simulink model "test_firs"  (Simulink 6.2)
settings: Solver=ode45  StartTime=0.0  StopTime=500  RelTol=1e-3
undefined symbols (not defined in the file or in its folder): now, pfb_coefs
libraries: xbsIndex_r3 x151, pfb_library x1, simulink x1
(part 1 of 3)
settings Model: LastModifiedBy=mdexter
settings DebuggingCC: SolverPrmCheckMsg=warning

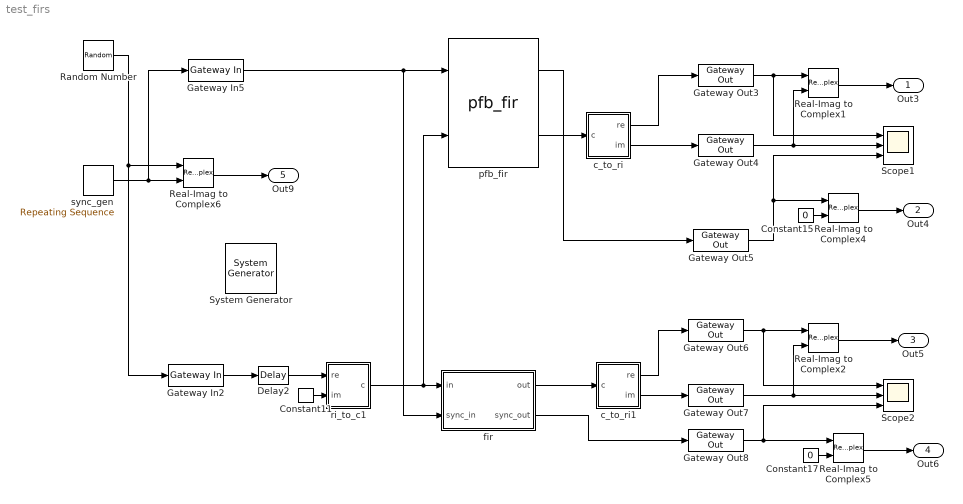
== system test_firs ==
  " System Generator" : xbsIndex_r3/ System Generator  Tag=genX  xilinxfamily=Virtex2  part=xc2v1000  speed=-4  package=bg575  synthesis_tool=XST  directory=./netlist  testbench=off  simulink_period=1  sysclk_period=100  incr_netlist=off  trim_vbits=Everywhere in SubSystem  dbl_ovrd=According to Block Masks  core_generation=According to Block Masks  run_coregen=off  deprecated_control=off  eval_field=0
      settings: AttributesFormatString=System\nGenerator
  Constant11 : xbsIndex_r3/Constant  const=0  equ=P=C  arith_type=Unsigned  n_bits=8  bin_pt=7  opselect=C  inp2=PCIN>>17  opr=+  inp1=P  carry=CIN  iostate=0  explicit_period=on  period=1  dbl_ovrd=off
  Constant15 : Constant  Value=0
  Constant17 : Constant  Value=0
  Delay2 : xbsIndex_r3/Delay  latency=1  reg_retiming=off  explicit_period=off  period=1  en=off  accept_only_valid=off  init_zero=on  dbl_ovrd=off  show_param=off
      settings: xl_area=[0, 0, 0, 0, 0, 0, 0]
  Gateway In2 : xbsIndex_r3/Gateway In  arith_type="Signed  (2's comp)"  n_bits=8  bin_pt=7  quantization="Round  (unbiased: +/- Inf)"  overflow=Wrap  period=1  timing_constraint=None  locs_specified=off  LOCs={}  needs_fixed_name=off  dbl_ovrd=off  show_param=off
      settings: xl_area=[0, 0, 0, 0, 0, 0, 0]
  Gateway In5 : xbsIndex_r3/Gateway In  arith_type=Boolean  n_bits=8  bin_pt=7  quantization=Truncate  overflow=Wrap  period=1  timing_constraint=None  locs_specified=off  LOCs={}  needs_fixed_name=off  dbl_ovrd=off  show_param=off
      settings: xl_area=[0, 0, 0, 0, 0, 0, 0]
  Gateway Out{3..8} (6 alike) : xbsIndex_r3/Gateway Out  output_type=Double  nbits=8  bin_pt=6  arith_type=Boolean  quantization=Truncate  overflow=Wrap  hdl_port=on  timing_constraint=None  locs_specified=off  LOCs={}  needs_fixed_name=off  show_param=off
      settings: xl_area=[0, 0, 0, 0, 0, 0, 0]
  Random Number : RandomNumber  Variance=.3^2  Seed=floor(100*(now-floor(now)))  SampleTime=1
  Real-Imag to Complex{1..2,4..6} (5 alike) : RealImagToComplex
  Scope1 : Scope  NumInputPorts=3
      settings: YMin=-5~-5~-5  YMax=5~5~5
  Scope2 : Scope  NumInputPorts=3
      settings: YMin=-5~-5~-5  YMax=5~5~5  SaveName=ScopeData2
  c_to_ri : Subsystem  mask(Complex to Real-Imag){n_bits=18, bin_pt=17}
      mask prompts: n_bits "Bit Width"; bin_pt "Binary Point"
      mask help: Outputs real and imaginary components of a complex input.
      mask init:
      | c_to_ri_init(gcb,n_bits,bin_pt);
      settings: AttributesFormatString=18_17 r/i
      mask Help:
      | <pre>
      | Description::
      | 
      | Outputs real and imaginary components of a complex input.
      | Useful for simplifying interconnects.
      | See also: Real-Imag to Complex (ri_to_c)
      | 
      | Mask Parameters::
      | 
      | Bit Width (n_bits): Specifies the width of the real/imaginary components.
      | Assumed equal for both components.
      | 
      | Binary Point (bin_pt): Specifies the binary point location in the real/imaginary components.
      | Assumed equal for both components.
      | </pre>
  c_to_ri1 : Subsystem  mask(Complex to Real-Imag){n_bits=9, bin_pt=7}
      mask prompts: n_bits "Bit Width"; bin_pt "Binary Point"
      mask help: Outputs real and imaginary components of a complex input.
      mask init:
      | c_to_ri_init(gcb,n_bits,bin_pt);
      settings: AttributesFormatString=9_7 r/i
      mask Help:
      | <pre>
      | Description::
      | 
      | Outputs real and imaginary components of a complex input.
      | Useful for simplifying interconnects.
      | See also: Real-Imag to Complex (ri_to_c)
      | 
      | Mask Parameters::
      | 
      | Bit Width (n_bits): Specifies the width of the real/imaginary components.
      | Assumed equal for both components.
      | 
      | Binary Point (bin_pt): Specifies the binary point location in the real/imaginary components.
      | Assumed equal for both components.
      | </pre>
  fir : Subsystem  AncestorBlock=newfft_library/FIR/fir  mask(FIR Filter){coefs=pfb_coefs(64,4), n_bits_c=9, bin_pt_c=8, n_bits_d=8, bin_pt_d=7, n_bits_o=9, bin_pt_o=7, coef_bram=on, delay_bram=on, mult_latency=3, add_latency=1, show_sbo=on, munge_submasks=DumbDown}
      mask prompts: coefs "Tap Coefficients"; n_bits_c "Number of Coefficient Bits"; bin_pt_c "Coefficient Binary Point"; n_bits_d "Number of Data Bits"; bin_pt_d "Data Binary Point"; n_bits_o "Number of Bits Out"; bin_pt_o "Binary Point Out"; coef_bram "Use BRAM for Coefficients"; delay_bram "Use BRAM for Delay"; mult_latency "Multiplier Latency"; add_latency "Adder Latency"; show_sbo "Show Sub-Block Options"; munge_submasks "Sub-Block Masks"
      mask help: A Finite Impluse Response Filter. This FIR filter does not have provisions for folding the input sequence to improve multiplier efficiency, so it is suboptimal for "regular" (i.e. non-WOLA) FIR filters. It is intended primarily for WOLA (Weighted OverLap Add) FIR filters.
      mask init:
      | tic
      | fir_init(gcb, ...
      |   coefs, ...
      |   n_bits_c, ...
      |   bin_pt_c, ...
      |   n_bits_d, ...
      |   bin_pt_d, ...
      |   n_bits_o, ...
      |   bin_pt_o, ...
      |   coef_bram, ...
      |   delay_bram, ...
      |   mult_latency, ...
      |   add_latency, ...
      |   lower(get_param(gcb,'munge_submasks')) );
      | disp('fir_init complete.');
      | toc
      settings: AttributesFormatString=|
      | 4 taps
      | 9_8 coefs
      | 8_7 in
      | 9_7 out
      mask Help:
      | <pre>
      | Description::
      | 
      | A Finite Impluse Response Filter.
      | 
      | This Finite Impluse Response Filter does not have provisions for folding the input
      | sequence to improve multiplier efficiency, so it is suboptimal for "regular" (i.e. non-WOLA)
      | FIR filters.  It is intended primarily for WOLA (Weighted OverLap Add) FIR filters.
      | 
      | Mask Parameters::
      | 
      | Coefficiant(s) (coefs): Matrix of real double(s) to use as coefficient(s).
      | One column per tap.  Multiple rows will create a WOLA filter.
      | These should be specified as doubles.  They will be rounded/saturated according to the
      | specified number of bits (n_bits_c) and binary point (bin_pt_c).
      | 
      | Number of Coefficient Bits (n_bits_c): The number of bits used for the fixed point binary
      | representation of the coefficient(s).
      | 
      | Coefficient Binary Point (bin_pt_c): The binary point of the fixed point binary representation
      | of the coefficient(s).
      | 
      | Number of Data Bits (n_bits_d): The number of bits for real/imaginary components of the data.
      | 
      | Data Binary Point (bin_pt_d): The binary point for real/imaginary components of the data.
      | 
      | Number of Bits Out (n_bits_o): Specifies the width of the output (overflow wraps).
      | The internal adders will use a bit width of (n_bits_o-bin_pt_o+bin_pt_c+bin_pt_d).
      | 
      | Binary Point Out (bin_pt_o): Specifies the binary point of the output (quantization truncates).
      | The internal adders will use a binary point of (bin_pt_c+bin_pt_d).
      | 
      | Use BRAM for Coefficients (coef_bram): Check this checkbox to store the coefficients in BRAM.
      | If unchecked, the coefficients will be stored in distributed memory (i.e. slices).
      | This is only relevant is length(coef) is greater than 1; otherwise, a constant block is used.
      | 
      | Use BRAM for Delay (delay_bram): Check this checkbox to implement the delay using BRAM.
      | If unchecked, the delay will be implemented using SLR16 elements (i.e. slices).
      | 
      | Multiplier Latency (mult_latency): Latency to use for the underlying multiplier.
      | 
      | Adder Latency (add_latency): Latency to use for the underlying adder.
      | </pre>
      mask StyleString: edit,edit,edit,edit,edit,edit,edit,checkbox,checkbox,edit,edit,checkbox,popup(Keep|DumbDown|Unmask)
      mask CallbackString:
      | |||||||||||mvs=get_param(gcb,'MaskVisibilityString');
      | if strcmp(get_param(gcb,'show_sbo'),'on')
      |   onoff='on';
      | else
      |   onoff='off';
      | end
      | mvs=regexprep(mvs,'o[nf]*$',onoff);
      | set_param(gcb,'MaskVisibilityString',mvs);
      | |
  pfb_fir : pfb_library/pfb_fir  PFBSize=6  TotalTaps=4  WindowType=hamming  n_inputs=0  MakeBiplex=off  BitWidthIn=8  BitWidthOut=18  CoeffBitWidth=9  CoeffDistMem=off  add_latency=1  mult_latency=3  bram_latency=1  quantization="Round  (unbiased: Even Values)"  fwidth=1
      link override pol1_in1_first_tap/sync_delay/Constant: equ=P=C
      link override pol1_in1_first_tap/sync_delay/Constant1: equ=P=C
      link override pol1_in1_first_tap/sync_delay/Constant2: equ=P=C
      link override pol1_in1_first_tap/sync_delay/Constant3: equ=P=C
      link override pol1_in1_tap2/sync_delay/Constant: equ=P=C
      link override pol1_in1_tap2/sync_delay/Constant1: equ=P=C
      link override pol1_in1_tap2/sync_delay/Constant2: equ=P=C
      link override pol1_in1_tap2/sync_delay/Constant3: equ=P=C
      link override pol1_in1_tap3/sync_delay/Constant: equ=P=C
      link override pol1_in1_tap3/sync_delay/Constant1: equ=P=C
      link override pol1_in1_tap3/sync_delay/Constant2: equ=P=C
      link override pol1_in1_tap3/sync_delay/Constant3: equ=P=C
  ri_to_c1 : Subsystem  mask(Real-Imag to Complex){}
      mask help: Concatenates real and imaginary inputs into a complex output.
      mask init:
      | ri_to_c_init(gcb);
      mask Help:
      | <pre>
      | Description::
      | 
      | Concatenates a real and imaginary input into a complex output.
      | Useful for simplifying interconnects.
      | See also: Complex to Real-Imag (c_to_ri)
      | 
      | Mask Parameters::
      | 
      | (N/A)
      | </pre>
  sync_gen : simulink/Sources/Repeating Sequence  rep_seq_t=[0:64]  rep_seq_y=[1 zeros(1,63) 1]
  Out3 : Outport
  Out4 : Outport  Port=2
  Out5 : Outport  Port=3
  Out6 : Outport  Port=4
  Out9 : Outport  Port=5
  wires:
  Random Number/1 -> Real-Imag to Complex6/1, Gateway In2/1
  Gateway Out3/1 -> Scope1/1, Real-Imag to Complex1/1
  Gateway Out4/1 -> Scope1/2, Real-Imag to Complex1/2
  Gateway Out5/1 -> Scope1/3, Real-Imag to Complex4/1
  Gateway In5/1 -> fir/2(sync_in), pfb_fir/1
  Gateway In2/1 -> Delay2/1
  Gateway Out6/1 -> Real-Imag to Complex2/1, Scope2/1
  Gateway Out7/1 -> Scope2/2, Real-Imag to Complex2/2
  Gateway Out8/1 -> Scope2/3, Real-Imag to Complex5/1
  fir/2(sync_out) -> Gateway Out8/1
  fir/1(out) -> c_to_ri1/1(c)
  c_to_ri/2(im) -> Gateway Out4/1
  ri_to_c1/1(c) -> fir/1(in), pfb_fir/2
  Constant11/1 -> ri_to_c1/2(im)
  sync_gen/1 -> Real-Imag to Complex6/2, Gateway In5/1
  Delay2/1 -> ri_to_c1/1(re)
  c_to_ri/1(re) -> Gateway Out3/1
  Real-Imag to Complex1/1 -> Out3/1
  c_to_ri1/1(re) -> Gateway Out6/1
  c_to_ri1/2(im) -> Gateway Out7/1
  Real-Imag to Complex2/1 -> Out5/1
  Real-Imag to Complex4/1 -> Out4/1
  Real-Imag to Complex5/1 -> Out6/1
  Constant15/1 -> Real-Imag to Complex4/2
  Constant17/1 -> Real-Imag to Complex5/2
  Real-Imag to Complex6/1 -> Out9/1
  pfb_fir/1 -> Gateway Out5/1
  pfb_fir/2 -> c_to_ri/1(c)

== system test_firs/c_to_ri ==
  c : Inport  Port=1  LatchInput=off
  force_im : xbsIndex_r3/Reinterpret  force_arith_type=on  arith_type="Signed  (2's comp)"  force_bin_pt=on  bin_pt=17  force_valid=on
  force_re : xbsIndex_r3/Reinterpret  force_arith_type=on  arith_type="Signed  (2's comp)"  force_bin_pt=on  bin_pt=17  force_valid=on
  slice_im : xbsIndex_r3/Slice  mode=Lower Bit Location + Width  nbits=18  bit1=0  base1=MSB of Input  bit0=0  base0=LSB of Input  boolean_output=off  explicit_period=off  period=1  dbl_ovrd=off
  slice_re : xbsIndex_r3/Slice  mode=Upper Bit Location + Width  nbits=18  bit1=0  base1=MSB of Input  bit0=0  base0=LSB of Input  boolean_output=off  explicit_period=off  period=1  dbl_ovrd=off
  re : Outport
  im : Outport  Port=2
  wires:
  slice_re/1 -> force_re/1
  slice_im/1 -> force_im/1
  force_re/1 -> re/1
  force_im/1 -> im/1
  c/1 -> slice_re/1, slice_im/1

== system test_firs/c_to_ri1 ==
  c : Inport  Port=1  LatchInput=off
  force_im : xbsIndex_r3/Reinterpret  force_arith_type=on  arith_type="Signed  (2's comp)"  force_bin_pt=on  bin_pt=7  force_valid=on
  force_re : xbsIndex_r3/Reinterpret  force_arith_type=on  arith_type="Signed  (2's comp)"  force_bin_pt=on  bin_pt=7  force_valid=on
  slice_im : xbsIndex_r3/Slice  mode=Lower Bit Location + Width  nbits=9  bit1=0  base1=MSB of Input  bit0=0  base0=LSB of Input  boolean_output=off  explicit_period=off  period=1  dbl_ovrd=off
  slice_re : xbsIndex_r3/Slice  mode=Upper Bit Location + Width  nbits=9  bit1=0  base1=MSB of Input  bit0=0  base0=LSB of Input  boolean_output=off  explicit_period=off  period=1  dbl_ovrd=off
  re : Outport
  im : Outport  Port=2
  wires:
  c/1 -> slice_im/1, slice_re/1
  force_im/1 -> im/1
  force_re/1 -> re/1
  slice_im/1 -> force_im/1
  slice_re/1 -> force_re/1

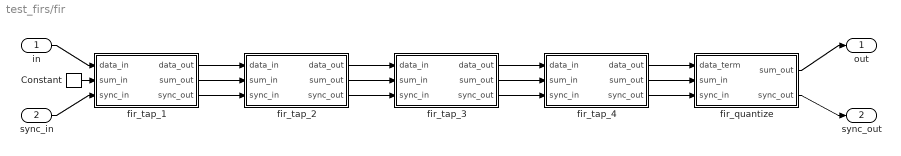
== system test_firs/fir ==
  in : Inport  Port=1  LatchInput=off
  sync_in : Inport  Port=2  LatchInput=off
  Constant : xbsIndex_r3/Constant  const=0  equ=P=C  arith_type=Unsigned  n_bits=34  bin_pt=0  opselect=C  inp2=PCIN>>17  opr=+  inp1=P  carry=CIN  iostate=0  explicit_period=on  period=1  dbl_ovrd=off
  fir_quantize : Subsystem  mask(FIR Filter Quantizer){n_bits_s=17, bin_pt_s=15, n_bits_o=9, bin_pt_o=7}
      mask prompts: n_bits_s "Number of Bits In"; bin_pt_s "Binary Point In"; n_bits_o "Number of Bits Out"; bin_pt_o "Binary Point Out"
      mask help: A Finite Impluse Response Filter ouput quantizer. This FIR filter output quantizer rounds the sum_in value to the precision specified by n_bits and bin_pt. Overflow wraps, but quantization rounds to even if input binary point is greater than output binary point, otherwise quantization tuncates.
      settings: AttributesFormatString=|
      | 17_15 in
      | 9_7 out
      | round even
      mask Help:
      | <pre>
      | Description::
      | 
      | A Finite Impluse Response Filter ouput quantizer.  This FIR filter output quantizer
      | rounds the sum_in value to the precision specified by n_bits and bin_pt.
      | 
      | Overflow wraps, but quantization rounds to even if input binary point is greater
      | than output binary point, otherwise quantization tuncates.
      | 
      | Mask Parameters::
      | 
      | Number of Bits In (n_bits_s): Specifies the width of the sum_in input.
      | 
      | Binary Point In (bin_pt_s): Specifies the binary point of the sum_in input.
      | 
      | Number of Bits Out (n_bits_o): Specifies the width of the output (overflow wraps).
      | 
      | Binary Point Out (bin_pt_o): Specifies the binary point of the output (quantization rounds to even
      | if input binary point is greater than output binary point, othersie quantization truncates).
      | </pre>
  fir_tap_1 : Subsystem  mask(FIR Filter Tap (Real Coefficients)){delay=64, coef=[-0.00411973909604202;-0.0119015518843096;-0.0190818823895147;-0.0256724955662416;-0.03168654178132;-0.0371384687203353;-0.0420439301426944;-0.0464196919199395;-0.0502835357982813;-0.0536541613305752;-0.0565510864251856;-0.0589945469593747;-0.0610053959030371;-0.0626050023947942;-0.0638151512067052;-0.0646579430261756;-0.0651556959741166;-0.0653308487670656;-0.0652058659179099;-0.064803145355121;-0.0641449288240917;-0.063253215416367;-0.0621496785533557;-0.0608555867306188;-0.0593917283071436;-0.057778340601254;-0.0560350435310833;-0.0541807780129703;-0.0522337493058552;-0.050211375463868;-0.0481302410329562;-0.0460060561007039;-0.0438536207815986;-0.0416867951930131;-0.039518474950235;-0.0373605721821118;-0.035224002042413;-0.0331186746659681;-0.0310534924931389;-0.0290363528613422;-0.0270741557382724;-0.0251728164482839;-0.0233372832211883;-0.0215715593716044;-0.0198787298970449;-0.018260992264242;-0.0167196911358607;-0.0152553567738119;-0.0138677468409146;-0.0125558913097251;-0.0113181401759998;-0.0101522136645361;-0.00905525460705801;-0.00802388266542662;-0.0070542500687595;-0.0061420985300509;-0.00528281700660057;-0.00447149996896613;-0.00370300584524142;-0.00297201531120363;-0.00227308910223182;-0.00160072502983972;-0.000949413894136895;-0.000313693993479576], n_bits_c=9, bin_pt_c=8, n_bits_d=8, bin_pt_d=7, n_bits_s=17, bin_pt_s=15, coef_bram=on, delay_bram=on, mult_latency=3, add_latency=1, add_bypass=on}
      mask prompts: delay "Tap Delay"; coef "Tap Coefficient(s)"; n_bits_c "Number of Coefficient Bits"; bin_pt_c "Coefficient Binary Point"; n_bits_d "Number of Data Bits"; bin_pt_d "Data Binary Point"; n_bits_s "Number of Sum Bits"; bin_pt_s "Sum Binary Point"; coef_bram "Use BRAM for Coefficients"; delay_bram "Use BRAM for Delay"; mult_latency "Multiplier Latency"; add_latency "Adder Latency"; add_bypass "Bypass Adder"
      mask help: A Finite Impluse Response Filter tap with real coefficients. This FIR filter tap does not have provisions for folding the input sequence to improve multiplier efficiency, so it is suboptimal for "regular" (i.e. non-WOLA) FIR filters. It is intended primarily for WOLA (Weighted OverLap Add) FIR filters.
      settings: AttributesFormatString=|
      | delay 64 in bram
      | 64 coefs in bram\nno adder
      mask Help:
      | <pre>
      | Description::
      | 
      | A Finite Impluse Response Filter tap with real coefficients.
      | 
      | This Finite Impluse Response Filter tap is designed to be daisy chained together
      | to form a multi-tap FIR filter.  This FIR filter tap does not have provisions for folding the input
      | sequence to improve multiplier efficiency, so it is suboptimal for "regular" (i.e. non-WOLA)
      | FIR filters.  It is intended primarily for WOLA (Weighted OverLap Add) FIR filters.
      | 
      | Mask Parameters::
      | 
      | Tap Delay (delay):  The inter-tap delay (the N in "z^-N").  For a regular FIR filter, this will be 1.
      | 
      | Tap Coefficiant(s) (coef): The coefficient(s) for this tap.  For a regular FIR filter, this will be a
      | single number.  For a WOLA (Weighted OverLap Add) filter, this will be a vector of numbers.
      | Usually, delay==length(coef), but this is not required.  These should be specified as doubles.
      | They will be rounded and saturated according to the specified number of bits (n_bits_c) and
      | binary point (bin_pt_c).
      | 
      | Number of Coefficient Bits (n_bits_c): The number of bits used for the fixed point binary
      | representation of the coefficient(s).
      | 
      | Coefficient Binary Point (bin_pt_c): The binary point of the fixed point binary representation
      | of the coefficient(s).
      | 
      | Number of Data Bits (n_bits_d): The number of bits for real/imaginary components of the data.
      | 
      | Data Binary Point (bin_pt_d): The binary point for real/imaginary components of the data.
      | 
      | Number of Sum Bits (n_bits_s): Specifies the width of the sum (overflow wraps).
      | 
      | Sum Binary Point (bin_pt_s): Specifies the binary point of the sum (quantization truncates).
      | 
      | Use BRAM for Delay (delay_bram): Check this checkbox to implement the delay using BRAM.
      | If unchecked, the delay will be implemented using SLR16 elements (i.e. slices).
      | 
      | Use BRAM for Coefficients (coef_bram): Check this checkbox to store the coefficients in BRAM.
      | If unchecked, the coefficients will be stored in distributed memory (i.e. slices).
      | This is only relevant is length(coef) is greater than 1; otherwise, a constant block is used.
      | 
      | Multiplier Latency (mult_latency): Latency to use for the underlying multiplier.
      | 
      | Adder Latency (add_latency): Latency to use for the underlying adder.
      | 
      | Adder Bypass (add_bypass): Check this checkbox to bypass the adder.
      | Typically used for the first tap of a multi-tap FIR filter.
      | </pre>
  fir_tap_2 : Subsystem  mask(FIR Filter Tap (Real Coefficients)){delay=64, coef=[0.999864698373715;0.998782787093866;0.996621638554108;0.993386591798817;0.989085632941254;0.983729368318744;0.977330988864374;0.969906225835535;0.961473298073597;0.952052851002189;0.941667887603872;0.93034369164628;0.918107743458883;0.904989628590384;0.891020939704144;0.876235172094917;0.860667613234385;0.844355226775522;0.827336531466419;0.809651475442971;0.791341306386551;0.772448438047459;0.75301631364748;0.733089266685254;0.712712379676312;0.691931341365526;0.670792302953398;0.649341733878935;0.627626277701018;0.605692608616936;0.58358728915143;0.561356629541902;0.539046549335732;0.516702441703681;0.494369040959443;0.47209029375942;0.449909234438953;0.427867864921515;0.406007039615979;0.384366355693955;0.362984049114638;0.341896896738581;0.321140124844505;0.300747324334799;0.280750372885839;0.261179364268877;0.242062545036048;0.22342625873426;0.205294897777456;0.187690863075115;0.170634531482069;0.154144231101832;0.138236224442934;0.122924699395207;0.108221767960864;0.0941374726436389;0.0806798003683017;0.0678547037727424;0.0556661296856254;0.0441160545744412;0.033204526721812;0.0229297148621999;0.0132879629868503;0.00427385100197821], n_bits_c=9, bin_pt_c=8, n_bits_d=8, bin_pt_d=7, n_bits_s=17, bin_pt_s=15, coef_bram=on, delay_bram=on, mult_latency=3, add_latency=1, add_bypass=off}
      mask prompts: delay "Tap Delay"; coef "Tap Coefficient(s)"; n_bits_c "Number of Coefficient Bits"; bin_pt_c "Coefficient Binary Point"; n_bits_d "Number of Data Bits"; bin_pt_d "Data Binary Point"; n_bits_s "Number of Sum Bits"; bin_pt_s "Sum Binary Point"; coef_bram "Use BRAM for Coefficients"; delay_bram "Use BRAM for Delay"; mult_latency "Multiplier Latency"; add_latency "Adder Latency"; add_bypass "Bypass Adder"
      mask help: A Finite Impluse Response Filter tap with real coefficients. This FIR filter tap does not have provisions for folding the input sequence to improve multiplier efficiency, so it is suboptimal for "regular" (i.e. non-WOLA) FIR filters. It is intended primarily for WOLA (Weighted OverLap Add) FIR filters.
      settings: AttributesFormatString=|
      | delay 64 in bram
      | 64 coefs in bram
      mask Help:
      | <pre>
      | Description::
      | 
      | A Finite Impluse Response Filter tap with real coefficients.
      | 
      | This Finite Impluse Response Filter tap is designed to be daisy chained together
      | to form a multi-tap FIR filter.  This FIR filter tap does not have provisions for folding the input
      | sequence to improve multiplier efficiency, so it is suboptimal for "regular" (i.e. non-WOLA)
      | FIR filters.  It is intended primarily for WOLA (Weighted OverLap Add) FIR filters.
      | 
      | Mask Parameters::
      | 
      | Tap Delay (delay):  The inter-tap delay (the N in "z^-N").  For a regular FIR filter, this will be 1.
      | 
      | Tap Coefficiant(s) (coef): The coefficient(s) for this tap.  For a regular FIR filter, this will be a
      | single number.  For a WOLA (Weighted OverLap Add) filter, this will be a vector of numbers.
      | Usually, delay==length(coef), but this is not required.  These should be specified as doubles.
      | They will be rounded and saturated according to the specified number of bits (n_bits_c) and
      | binary point (bin_pt_c).
      | 
      | Number of Coefficient Bits (n_bits_c): The number of bits used for the fixed point binary
      | representation of the coefficient(s).
      | 
      | Coefficient Binary Point (bin_pt_c): The binary point of the fixed point binary representation
      | of the coefficient(s).
      | 
      | Number of Data Bits (n_bits_d): The number of bits for real/imaginary components of the data.
      | 
      | Data Binary Point (bin_pt_d): The binary point for real/imaginary components of the data.
      | 
      | Number of Sum Bits (n_bits_s): Specifies the width of the sum (overflow wraps).
      | 
      | Sum Binary Point (bin_pt_s): Specifies the binary point of the sum (quantization truncates).
      | 
      | Use BRAM for Delay (delay_bram): Check this checkbox to implement the delay using BRAM.
      | If unchecked, the delay will be implemented using SLR16 elements (i.e. slices).
      | 
      | Use BRAM for Coefficients (coef_bram): Check this checkbox to store the coefficients in BRAM.
      | If unchecked, the coefficients will be stored in distributed memory (i.e. slices).
      | This is only relevant is length(coef) is greater than 1; otherwise, a constant block is used.
      | 
      | Multiplier Latency (mult_latency): Latency to use for the underlying multiplier.
      | 
      | Adder Latency (add_latency): Latency to use for the underlying adder.
      | 
      | Adder Bypass (add_bypass): Check this checkbox to bypass the adder.
      | Typically used for the first tap of a multi-tap FIR filter.
      | </pre>
  fir_tap_3 : Subsystem  mask(FIR Filter Tap (Real Coefficients)){delay=64, coef=[0.00427385100197821;0.0132879629868503;0.0229297148621999;0.033204526721812;0.0441160545744412;0.0556661296856254;0.0678547037727424;0.0806798003683017;0.0941374726436389;0.108221767960864;0.122924699395207;0.138236224442934;0.154144231101832;0.170634531482069;0.187690863075115;0.205294897777456;0.22342625873426;0.242062545036048;0.261179364268877;0.280750372885839;0.300747324334799;0.321140124844505;0.341896896738581;0.362984049114638;0.384366355693955;0.406007039615979;0.427867864921515;0.449909234438953;0.47209029375942;0.494369040959443;0.516702441703681;0.539046549335732;0.561356629541902;0.58358728915143;0.605692608616936;0.627626277701018;0.649341733878935;0.670792302953398;0.691931341365526;0.712712379676312;0.733089266685254;0.75301631364748;0.772448438047459;0.791341306386551;0.809651475442971;0.827336531466419;0.844355226775522;0.860667613234385;0.876235172094917;0.891020939704144;0.904989628590384;0.918107743458883;0.93034369164628;0.941667887603872;0.952052851002189;0.961473298073597;0.969906225835535;0.977330988864374;0.983729368318744;0.989085632941254;0.993386591798817;0.996621638554108;0.998782787093866;0.999864698373715], n_bits_c=9, bin_pt_c=8, n_bits_d=8, bin_pt_d=7, n_bits_s=17, bin_pt_s=15, coef_bram=on, delay_bram=on, mult_latency=3, add_latency=1, add_bypass=off}
      mask prompts: delay "Tap Delay"; coef "Tap Coefficient(s)"; n_bits_c "Number of Coefficient Bits"; bin_pt_c "Coefficient Binary Point"; n_bits_d "Number of Data Bits"; bin_pt_d "Data Binary Point"; n_bits_s "Number of Sum Bits"; bin_pt_s "Sum Binary Point"; coef_bram "Use BRAM for Coefficients"; delay_bram "Use BRAM for Delay"; mult_latency "Multiplier Latency"; add_latency "Adder Latency"; add_bypass "Bypass Adder"
      mask help: A Finite Impluse Response Filter tap with real coefficients. This FIR filter tap does not have provisions for folding the input sequence to improve multiplier efficiency, so it is suboptimal for "regular" (i.e. non-WOLA) FIR filters. It is intended primarily for WOLA (Weighted OverLap Add) FIR filters.
      settings: AttributesFormatString=|
      | delay 64 in bram
      | 64 coefs in bram
      mask Help:
      | <pre>
      | Description::
      | 
      | A Finite Impluse Response Filter tap with real coefficients.
      | 
      | This Finite Impluse Response Filter tap is designed to be daisy chained together
      | to form a multi-tap FIR filter.  This FIR filter tap does not have provisions for folding the input
      | sequence to improve multiplier efficiency, so it is suboptimal for "regular" (i.e. non-WOLA)
      | FIR filters.  It is intended primarily for WOLA (Weighted OverLap Add) FIR filters.
      | 
      | Mask Parameters::
      | 
      | Tap Delay (delay):  The inter-tap delay (the N in "z^-N").  For a regular FIR filter, this will be 1.
      | 
      | Tap Coefficiant(s) (coef): The coefficient(s) for this tap.  For a regular FIR filter, this will be a
      | single number.  For a WOLA (Weighted OverLap Add) filter, this will be a vector of numbers.
      | Usually, delay==length(coef), but this is not required.  These should be specified as doubles.
      | They will be rounded and saturated according to the specified number of bits (n_bits_c) and
      | binary point (bin_pt_c).
      | 
      | Number of Coefficient Bits (n_bits_c): The number of bits used for the fixed point binary
      | representation of the coefficient(s).
      | 
      | Coefficient Binary Point (bin_pt_c): The binary point of the fixed point binary representation
      | of the coefficient(s).
      | 
      | Number of Data Bits (n_bits_d): The number of bits for real/imaginary components of the data.
      | 
      | Data Binary Point (bin_pt_d): The binary point for real/imaginary components of the data.
      | 
      | Number of Sum Bits (n_bits_s): Specifies the width of the sum (overflow wraps).
      | 
      | Sum Binary Point (bin_pt_s): Specifies the binary point of the sum (quantization truncates).
      | 
      | Use BRAM for Delay (delay_bram): Check this checkbox to implement the delay using BRAM.
      | If unchecked, the delay will be implemented using SLR16 elements (i.e. slices).
      | 
      | Use BRAM for Coefficients (coef_bram): Check this checkbox to store the coefficients in BRAM.
      | If unchecked, the coefficients will be stored in distributed memory (i.e. slices).
      | This is only relevant is length(coef) is greater than 1; otherwise, a constant block is used.
      | 
      | Multiplier Latency (mult_latency): Latency to use for the underlying multiplier.
      | 
      | Adder Latency (add_latency): Latency to use for the underlying adder.
      | 
      | Adder Bypass (add_bypass): Check this checkbox to bypass the adder.
      | Typically used for the first tap of a multi-tap FIR filter.
      | </pre>
  fir_tap_4 : Subsystem  mask(FIR Filter Tap (Real Coefficients)){delay=0, coef=[-0.000313693993479576;-0.000949413894136895;-0.00160072502983972;-0.00227308910223182;-0.00297201531120363;-0.00370300584524142;-0.00447149996896613;-0.00528281700660057;-0.0061420985300509;-0.0070542500687595;-0.00802388266542662;-0.00905525460705801;-0.0101522136645361;-0.0113181401759998;-0.0125558913097251;-0.0138677468409146;-0.0152553567738119;-0.0167196911358607;-0.018260992264242;-0.0198787298970449;-0.0215715593716044;-0.0233372832211883;-0.0251728164482839;-0.0270741557382724;-0.0290363528613422;-0.0310534924931389;-0.0331186746659681;-0.035224002042413;-0.0373605721821118;-0.039518474950235;-0.0416867951930131;-0.0438536207815986;-0.0460060561007039;-0.0481302410329562;-0.050211375463868;-0.0522337493058552;-0.0541807780129703;-0.0560350435310833;-0.057778340601254;-0.0593917283071436;-0.0608555867306188;-0.0621496785533557;-0.063253215416367;-0.0641449288240917;-0.064803145355121;-0.0652058659179099;-0.0653308487670656;-0.0651556959741166;-0.0646579430261756;-0.0638151512067052;-0.0626050023947942;-0.0610053959030371;-0.0589945469593747;-0.0565510864251856;-0.0536541613305752;-0.0502835357982813;-0.0464196919199395;-0.0420439301426944;-0.0371384687203353;-0.03168654178132;-0.0256724955662416;-0.0190818823895147;-0.0119015518843096;-0.00411973909604202], n_bits_c=9, bin_pt_c=8, n_bits_d=8, bin_pt_d=7, n_bits_s=17, bin_pt_s=15, coef_bram=on, delay_bram=off, mult_latency=3, add_latency=1, add_bypass=off}
      mask prompts: delay "Tap Delay"; coef "Tap Coefficient(s)"; n_bits_c "Number of Coefficient Bits"; bin_pt_c "Coefficient Binary Point"; n_bits_d "Number of Data Bits"; bin_pt_d "Data Binary Point"; n_bits_s "Number of Sum Bits"; bin_pt_s "Sum Binary Point"; coef_bram "Use BRAM for Coefficients"; delay_bram "Use BRAM for Delay"; mult_latency "Multiplier Latency"; add_latency "Adder Latency"; add_bypass "Bypass Adder"
      mask help: A Finite Impluse Response Filter tap with real coefficients. This FIR filter tap does not have provisions for folding the input sequence to improve multiplier efficiency, so it is suboptimal for "regular" (i.e. non-WOLA) FIR filters. It is intended primarily for WOLA (Weighted OverLap Add) FIR filters.
      settings: AttributesFormatString=|
      | delay 0 in slr
      | 64 coefs in bram
      mask Help:
      | <pre>
      | Description::
      | 
      | A Finite Impluse Response Filter tap with real coefficients.
      | 
      | This Finite Impluse Response Filter tap is designed to be daisy chained together
      | to form a multi-tap FIR filter.  This FIR filter tap does not have provisions for folding the input
      | sequence to improve multiplier efficiency, so it is suboptimal for "regular" (i.e. non-WOLA)
      | FIR filters.  It is intended primarily for WOLA (Weighted OverLap Add) FIR filters.
      | 
      | Mask Parameters::
      | 
      | Tap Delay (delay):  The inter-tap delay (the N in "z^-N").  For a regular FIR filter, this will be 1.
      | 
      | Tap Coefficiant(s) (coef): The coefficient(s) for this tap.  For a regular FIR filter, this will be a
      | single number.  For a WOLA (Weighted OverLap Add) filter, this will be a vector of numbers.
      | Usually, delay==length(coef), but this is not required.  These should be specified as doubles.
      | They will be rounded and saturated according to the specified number of bits (n_bits_c) and
      | binary point (bin_pt_c).
      | 
      | Number of Coefficient Bits (n_bits_c): The number of bits used for the fixed point binary
      | representation of the coefficient(s).
      | 
      | Coefficient Binary Point (bin_pt_c): The binary point of the fixed point binary representation
      | of the coefficient(s).
      | 
      | Number of Data Bits (n_bits_d): The number of bits for real/imaginary components of the data.
      | 
      | Data Binary Point (bin_pt_d): The binary point for real/imaginary components of the data.
      | 
      | Number of Sum Bits (n_bits_s): Specifies the width of the sum (overflow wraps).
      | 
      | Sum Binary Point (bin_pt_s): Specifies the binary point of the sum (quantization truncates).
      | 
      | Use BRAM for Delay (delay_bram): Check this checkbox to implement the delay using BRAM.
      | If unchecked, the delay will be implemented using SLR16 elements (i.e. slices).
      | 
      | Use BRAM for Coefficients (coef_bram): Check this checkbox to store the coefficients in BRAM.
      | If unchecked, the coefficients will be stored in distributed memory (i.e. slices).
      | This is only relevant is length(coef) is greater than 1; otherwise, a constant block is used.
      | 
      | Multiplier Latency (mult_latency): Latency to use for the underlying multiplier.
      | 
      | Adder Latency (add_latency): Latency to use for the underlying adder.
      | 
      | Adder Bypass (add_bypass): Check this checkbox to bypass the adder.
      | Typically used for the first tap of a multi-tap FIR filter.
      | </pre>
  out : Outport
  sync_out : Outport  Port=2
  wires:
  in/1 -> fir_tap_1/1(data_in)
  sync_in/1 -> fir_tap_1/3(sync_in)
  fir_tap_1/1(data_out) -> fir_tap_2/1(data_in)
  fir_tap_1/2(sum_out) -> fir_tap_2/2(sum_in)
  fir_tap_1/3(sync_out) -> fir_tap_2/3(sync_in)
  fir_tap_2/1(data_out) -> fir_tap_3/1(data_in)
  fir_tap_2/2(sum_out) -> fir_tap_3/2(sum_in)
  fir_tap_2/3(sync_out) -> fir_tap_3/3(sync_in)
  fir_tap_3/1(data_out) -> fir_tap_4/1(data_in)
  fir_tap_3/2(sum_out) -> fir_tap_4/2(sum_in)
  fir_tap_3/3(sync_out) -> fir_tap_4/3(sync_in)
  fir_tap_4/1(data_out) -> fir_quantize/1(data_term)
  fir_tap_4/2(sum_out) -> fir_quantize/2(sum_in)
  fir_tap_4/3(sync_out) -> fir_quantize/3(sync_in)
  fir_quantize/1(sum_out) -> out/1
  fir_quantize/2(sync_out) -> sync_out/1
  Constant/1 -> fir_tap_1/2(sum_in)

== system test_firs/ri_to_c1 ==
  re : Inport  Port=1  LatchInput=off
  im : Inport  Port=2  LatchInput=off
  concat : xbsIndex_r3/Concat  num_inputs=2  explicit_period=off  period=1  dbl_ovrd=off
  force_im : xbsIndex_r3/Reinterpret  force_arith_type=on  arith_type=Unsigned  force_bin_pt=on  bin_pt=0  force_valid=on
  force_re : xbsIndex_r3/Reinterpret  force_arith_type=on  arith_type=Unsigned  force_bin_pt=on  bin_pt=0  force_valid=on
  c : Outport
  wires:
  im/1 -> force_im/1
  concat/1 -> c/1
  re/1 -> force_re/1
  force_im/1 -> concat/2
  force_re/1 -> concat/1

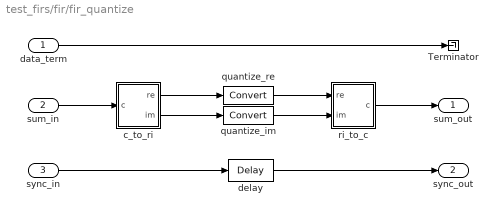
== system test_firs/fir/fir_quantize ==
  data_term : Inport  Port=1  LatchInput=off
  sum_in : Inport  Port=2  LatchInput=off
  sync_in : Inport  Port=3  LatchInput=off
  Terminator : Terminator
  c_to_ri : Subsystem  mask(Complex to Real-Imag){n_bits=17, bin_pt=15}
      mask prompts: n_bits "Bit Width"; bin_pt "Binary Point"
      mask help: Outputs real and imaginary components of a complex input.
      settings: AttributesFormatString=17_15 r/i
      mask Help:
      | <pre>
      | Description::
      | 
      | Outputs real and imaginary components of a complex input.
      | Useful for simplifying interconnects.
      | See also: Real-Imag to Complex (ri_to_c)
      | 
      | Mask Parameters::
      | 
      | Bit Width (n_bits): Specifies the width of the real/imaginary components.
      | Assumed equal for both components.
      | 
      | Binary Point (bin_pt): Specifies the binary point location in the real/imaginary components.
      | Assumed equal for both components.
      | </pre>
  delay : xbsIndex_r3/Delay  latency=3  reg_retiming=off  explicit_period=off  period=1  en=off  accept_only_valid=off  init_zero=on  dbl_ovrd=off  show_param=on
      settings: xl_area=[0, 0, 0, 0, 0, 0, 0]
  quantize_im : xbsIndex_r3/Convert  arith_type="Signed  (2's comp)"  n_bits=9  bin_pt=7  quantization="Round  (unbiased: Even Values)"  overflow=Wrap  latency=3  explicit_period=off  period=1  dbl_ovrd=off  show_param=on  inserted_by_tool=off  pipeline=on
      settings: xl_area=[0, 0, 0, 0, 0, 0, 0]
  quantize_re : xbsIndex_r3/Convert  arith_type="Signed  (2's comp)"  n_bits=9  bin_pt=7  quantization="Round  (unbiased: Even Values)"  overflow=Wrap  latency=3  explicit_period=off  period=1  dbl_ovrd=off  show_param=on  inserted_by_tool=off  pipeline=on
      settings: xl_area=[0, 0, 0, 0, 0, 0, 0]
  ri_to_c : Subsystem  mask(Real-Imag to Complex){}
      mask help: Concatenates real and imaginary inputs into a complex output.
      mask init:
      | ri_to_c_init(gcb);
      mask Help:
      | <pre>
      | Description::
      | 
      | Concatenates a real and imaginary input into a complex output.
      | Useful for simplifying interconnects.
      | See also: Complex to Real-Imag (c_to_ri)
      | 
      | Mask Parameters::
      | 
      | (N/A)
      | </pre>
  sum_out : Outport
  sync_out : Outport  Port=2
  wires:
  data_term/1 -> Terminator/1
  delay/1 -> sync_out/1
  sync_in/1 -> delay/1
  quantize_im/1 -> ri_to_c/2(im)
  c_to_ri/2(im) -> quantize_im/1
  quantize_re/1 -> ri_to_c/1(re)
  c_to_ri/1(re) -> quantize_re/1
  ri_to_c/1(c) -> sum_out/1
  sum_in/1 -> c_to_ri/1(c)

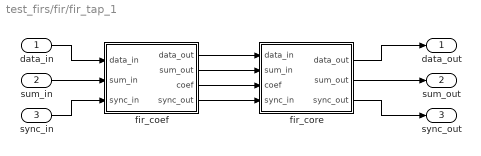
== system test_firs/fir/fir_tap_1 ==
  data_in : Inport  Port=1  LatchInput=off
  sum_in : Inport  Port=2  LatchInput=off
  sync_in : Inport  Port=3  LatchInput=off
  fir_coef : Subsystem  mask(FIR Filter Coefficient Generator){coef=[-0.00411973909604202;-0.0119015518843096;-0.0190818823895147;-0.0256724955662416;-0.03168654178132;-0.0371384687203353;-0.0420439301426944;-0.0464196919199395;-0.0502835357982813;-0.0536541613305752;-0.0565510864251856;-0.0589945469593747;-0.0610053959030371;-0.0626050023947942;-0.0638151512067052;-0.0646579430261756;-0.0651556959741166;-0.0653308487670656;-0.0652058659179099;-0.064803145355121;-0.0641449288240917;-0.063253215416367;-0.0621496785533557;-0.0608555867306188;-0.0593917283071436;-0.057778340601254;-0.0560350435310833;-0.0541807780129703;-0.0522337493058552;-0.050211375463868;-0.0481302410329562;-0.0460060561007039;-0.0438536207815986;-0.0416867951930131;-0.039518474950235;-0.0373605721821118;-0.035224002042413;-0.0331186746659681;-0.0310534924931389;-0.0290363528613422;-0.0270741557382724;-0.0251728164482839;-0.0233372832211883;-0.0215715593716044;-0.0198787298970449;-0.018260992264242;-0.0167196911358607;-0.0152553567738119;-0.0138677468409146;-0.0125558913097251;-0.0113181401759998;-0.0101522136645361;-0.00905525460705801;-0.00802388266542662;-0.0070542500687595;-0.0061420985300509;-0.00528281700660057;-0.00447149996896613;-0.00370300584524142;-0.00297201531120363;-0.00227308910223182;-0.00160072502983972;-0.000949413894136895;-0.000313693993479576], n_bits_c=9, bin_pt_c=8, use_bram=on}
      mask prompts: coef "Tap Coefficient(s)"; n_bits_c "Number of Coefficient Bits"; bin_pt_c "Coefficient Binary Point"; use_bram "Use BRAM for Coefficients"
      mask help: A Finite Impluse Response filter coefficient generator. This FIR filter coefficient generator outputs real coefficients. It can output one coefficient or cycle through a vector of coefficients for WOLA (Weighted OverLap Add) FIR filters.
      settings: AttributesFormatString=64 coefs in bram
      mask Help:
      | <pre>
      | Description::
      | 
      | A Finite Impluse Response filter coefficient generator.
      | This FIR filter coefficient generator outputs real coefficients.
      | It can output one coefficient or cycle through a vector of coefficients for WOLA
      | (Weighted OverLap Add) FIR filters.
      | 
      | Mask Parameters::
      | 
      | Tap Coefficiant(s) (coef): The coefficient(s) to output.  For a "regular" FIR filter, this will be a
      | single number.  For a WOLA (Weighted OverLap Add) filter, this will be a vector of numbers.
      | These should be specified as doubles.   They will be rounded and saturated according to the
      | specified number of bits (n_bits_c) and binary point (bin_pt_c).
      | 
      | Number of Coefficient Bits (n_bits_c): The number of bits used for the fixed point binary
      | representation of the coefficient(s).
      | 
      | Coefficient Binary Point (bin_pt_c): The binary point of the fixed point binary representation
      | of the coefficient(s).
      | 
      | Use BRAM for Coefficients (use_bram): Check this checkbox to store the coefficients in BRAM.
      | If unchecked, the coefficients will be stored in distributed memory (i.e. slices).
      | This is only relevant is length(coef) is greater than 1; otherwise, a constant block is used.
      | </pre>
  fir_core : Subsystem  mask(FIR Filter Core){delay=64, n_bits_d=8, bin_pt_d=7, n_bits_s=17, bin_pt_s=15, use_bram=on, mult_latency=3, add_latency=1, add_bypass=on}
      mask prompts: delay "Tap Delay"; n_bits_d "Number of Data Bits"; bin_pt_d "Data Binary Point"; n_bits_s "Number of Sum Bits"; bin_pt_s "Sum Binary Point"; use_bram "Use BRAM for Delay"; mult_latency "Multiplier Latency"; add_latency "Adder Latency"; add_bypass "Bypass Adder"
      mask help: A Finite Impluse Response Filter core with complex inputs and real coefficients. This FIR filter core does not have provisions for folding the input sequence to improve multiplier efficiency, so it is suboptimal for "regular" (i.e. non-WOLA) FIR filters. It is intended primarily for WOLA (Weighted OverLap Add) FIR filters.
      settings: AttributesFormatString=delay 64 in bram\nno adder
      mask Help:
      | <pre>
      | Description::
      | 
      | A Finite Impluse Response Filter core with complex inputs and real coefficients.
      | 
      | This Finite Impluse Response Filter core is designed to be paired with a FIR Coefficient Generator
      | to form a FIR filter tap.  This FIR filter core does not have provisions for folding the input
      | sequence to improve multiplier efficiency, so it is suboptimal for "regular" (i.e. non-WOLA)
      | FIR filters.  It is intended primarily for WOLA (Weighted OverLap Add) FIR filters.
      | 
      | Mask Parameters::
      | 
      | Tap Delay (delay):  The inter-tap delay (the N in "z^-N").  For a regular FIR filter, this will be 1.
      | 
      | Number of Data Bits (n_bits_d): The number of bits for real/imaginary components of the data.
      | 
      | Data Binary Point (bin_pt_d): The binary point for real/imaginary components of the data.
      | 
      | Number of Sum Bits (n_bits_s): Specifies the width of the sum (overflow wraps).
      | 
      | Sum Binary Point (bin_pt_s): Specifies the binary point of the sum (quantization truncates).
      | 
      | Use BRAM for Delay (use_bram): Check this checkbox to implement the delay using BRAM.
      | If unchecked, the delay will be implemented using SLR16 elements (i.e. slices).
      | 
      | Multiplier Latency (mult_latency): Latency to use for the underlying multiplier.
      | 
      | Adder Latency (add_latency): Latency to use for the underlying adder.
      | 
      | Adder Bypass (add_bypass): Check this checkbox to bypass the adder.
      | Typically used for the first tap of a multi-tap FIR filter.
      | </pre>
  data_out : Outport
  sum_out : Outport  Port=2
  sync_out : Outport  Port=3
  wires:
  fir_core/3(sync_out) -> sync_out/1
  fir_core/2(sum_out) -> sum_out/1
  fir_core/1(data_out) -> data_out/1
  sync_in/1 -> fir_coef/3(sync_in)
  sum_in/1 -> fir_coef/2(sum_in)
  data_in/1 -> fir_coef/1(data_in)
  fir_coef/4(sync_out) -> fir_core/4(sync_in)
  fir_coef/3(coef) -> fir_core/3(coef)
  fir_coef/2(sum_out) -> fir_core/2(sum_in)
  fir_coef/1(data_out) -> fir_core/1(data_in)
